simulink library "powermode"  (R2015b)
settings: Solver=ode1  StartTime=0.0  StopTime=Inf  FixedStep=0.001  RelTol=1e-3
PostLoadFcn:
  | , if any(exist('dsrtsu_mdlpostloadfcn', 'file') == [2, 3, 6]), try dsrtsu_mdlpostloadfcn('Execute', bdroot); catch fprintf('Error in PostLoadFcn (dsrtsu_mdlpostloadfcn) for model "%s":\n %s\n', bdroot, lasterr); end, end,
settings Model: DSRTSU_INTERNAL_RTI_VER=460  DSRTSU_INTERNAL_RTI_TYPE=rti1401  DSRTSU_INTERNAL_RTIFPGA=50  Creator=luis  LastModifiedBy=luis
settings OptimizationCC: BlockReduction=off  OptimizeBlockIOStorage=off  BufferReuse=off  GlobalBufferReuse=off  ExpressionFolding=off  LocalBlockOutputs=off
settings HardwareCC: ProdEndianess=BigEndian  ProdWordSize=32  ProdHWDeviceType=Generic->Custom  TargetIntDivRoundTo=Zero  TargetEndianess=BigEndian  TargetHWDeviceType=Generic->Custom
settings RTWCC: SystemTargetFile=rti1401.tlc  MakeCommand=make_rti  TemplateMakefile=rti1401.tmf  Description=dSPACE DS1401 Hardware Platform
settings STFCustomTargetCC: ParMdlRefBuildCompliant=on  ConcurrentExecutionCompliant=off  GeneratePreprocessorConditionals=Use local settings  MatFileLogging=on  CPPClassGenCompliant=off  SystemTargetFile=rti1401.tlc
settings GRTTargetCC: CompOptLevelCompliant=off  ConcurrentExecutionCompliant=off  CombineOutputUpdateFcns=off  CPPClassGenCompliant=off  GRTInterface=on  UseToolchainInfoCompliant=off  ExtModeMexFile=noextcomm

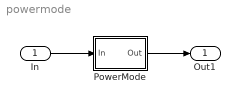
== system powermode ==
  In : Inport
  PowerMode : Subsystem
  Out1 : Outport
  wires:
  In/1 -> PowerMode/1(In)
  PowerMode/1(Out) -> Out1/1

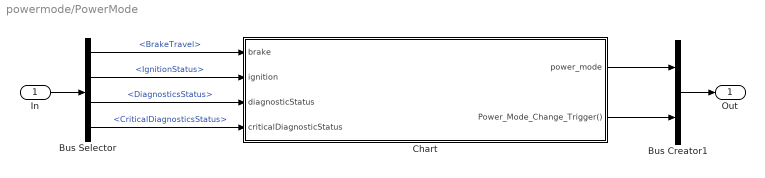
== system powermode/PowerMode ==
  In : Inport
  Bus Creator1 : BusCreator  Inputs=2
  Bus Selector : BusSelector  OutputSignals=BrakeTravel,IgnitionStatus,DiagnosticsStatus,CriticalDiagnosticsStatus
  Chart : Stateflow chart  TreatAsAtomicUnit=on
  Out : Outport
  wires:
  Chart/2(Power_Mode_Change_Trigger()) -> Bus Creator1/2
  Bus Selector/4 -> Chart/4(criticalDiagnosticStatus)  "<CriticalDiagnosticsStatus>"
  Bus Selector/2 -> Chart/2(ignition)  "<IgnitionStatus>"
  Bus Selector/3 -> Chart/3(diagnosticStatus)  "<DiagnosticsStatus>"
  In/1 -> Bus Selector/1
  Chart/1(power_mode) -> Bus Creator1/1
  Bus Creator1/1 -> Out/1
  Bus Selector/1 -> Chart/1(brake)  "<BrakeTravel>"

== stateflow chart powermode/PowerMode/Chart ==
  state Startup
    entry:
    power_mode = PowerModes.StartUp;
    Power_Mode_Change_Trigger();
    during:
    exit:
  state Idle
    entry:
    power_mode = PowerModes.Idle;
    Power_Mode_Change_Trigger();
    during:
    exit:
  state PreRTD
  state ReadyToDrive
    entry:
    power_mode = PowerModes.RTD;
    Power_Mode_Change_Trigger();
    during:
    exit:
  note: Non critical fault
      | Recovered
  state Stopped
    entry:
    power_mode = PowerModes.Stopped;
    Power_Mode_Change_Trigger();
    during:
    exit:
  state Fault
    entry:
    power_mode = PowerModes.Faulted;
    Power_Mode_Change_Trigger();
    during:
    exit:
  note: Critical Fault
      | Detected
  note: Fault
      | Detected
  (default) -> Startup
  Startup -> Idle : after(2,sec)
  Idle -> PreRTD [order 2] : [brake > 90 && ignition == 0]
  PreRTD -> ReadyToDrive [order 2] : [ignition == 1]
  PreRTD -> Idle [order 1] : [brake < 90 || diagnosticStatus == 1 || criticalDiagnosticStatus == 1]
  ReadyToDrive -> Idle [order 2] : [ignition == 0]
  ReadyToDrive -> Fault [order 1] : [diagnosticStatus == 1 || criticalDiagnosticStatus == 1]
  Fault -> ReadyToDrive [order 2] : [diagnosticStatus ~= 1 ]
  Idle -> Stopped [order 1] : [diagnosticStatus == 1 || criticalDiagnosticStatus == 1]
  Stopped -> Idle : [diagnosticStatus ~= 1 && criticalDiagnosticStatus ~= 1]
  Fault -> Stopped [order 1] : [criticalDiagnosticStatus == 1]
  data: power_mode output Enum: PowerModes =PowerModes.Undefined; brake input [0..100]; ignition input; diagnosticStatus input; criticalDiagnosticStatus input
  events: Power_Mode_Change_Trigger output FUNCTION_CALL_EVENT
